simulink model "DEF_IEEE14_case2"  (R2022b)
settings: Solver=FixedStepAuto  StartTime=0  StopTime=60  FixedStep=Ts  RelTol=1e-3
StopFcn:
  | data_idq_all_case2 = out.data_idq_all_case2;
  | save('Oscillation_July\data\data_idq_all_case2.mat','data_idq_all_case2');
  | data_vdq_all_case2 = out.data_vdq_all_case2;
  | save('Oscillation_July\data\data_vdq_all_case2.mat','data_vdq_all_case2');
undefined symbols (not defined in the file or in its folder): ApparatusDiscreDamping, ApparatusPara, ApparatusPowerFlow, ApparatusType, Fbase, OtherInputs, Sbase, Ts, Vbase, Wbase, x_e, Ybase, Zbase
libraries: spsGroundLib x22, SimplusGT x22, spsThreePhaseSeriesRLCBranchLib x20, spsThreePhaseParallelRLCBranchLib x14, spsabctoAlphaBetaZeroLib x8, spsThreePhaseTransformerTwoWindingsLib x3, spspowerguiLib x1
(part 1 of 2)
settings Model: LastModifiedBy=y_zhu

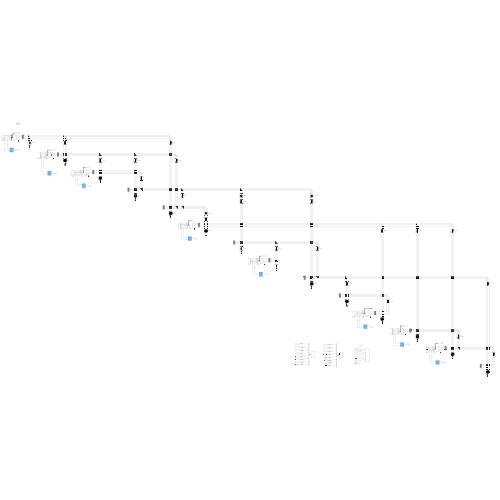
[thumbnail: Simulink's stored preview of the top-level diagram]
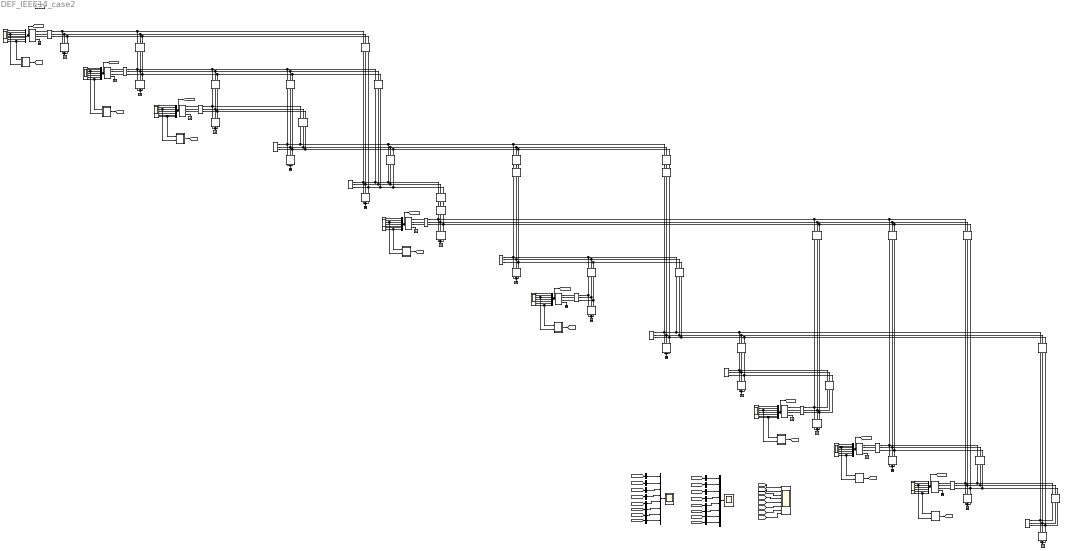
== system DEF_IEEE14_case2 ==
  note: DEF METHOD
  B-GND{1,4,8,10,14,16,20,23..24,27,29..30,32,34} (14 alike) : spsGroundLib/Ground  LConnTagsString=a
  Branch1-1 : spsThreePhaseParallelRLCBranchLib/Three-Phase Parallel RLC Branch  LConnTagsString=A|B|C  RConnTagsString=A|B|C  BranchType=C  Resistance=(Inf)*Zbase  Inductance=(Inf)*Zbase/Wbase  Capacitance=(0.051)*Ybase/Wbase  Measurements=None
  Branch1-2 : spsThreePhaseSeriesRLCBranchLib/Three-Phase Series RLC Branch  LConnTagsString=A|B|C  RConnTagsString=A|B|C  BranchType=RL  Resistance=(0.01938)*Zbase  Inductance=(0.05917)*Zbase/Wbase  Capacitance=1e-6  Measurements=None
  Branch1-5 : spsThreePhaseSeriesRLCBranchLib/Three-Phase Series RLC Branch  LConnTagsString=A|B|C  RConnTagsString=A|B|C  BranchType=RL  Resistance=(0.05403)*Zbase  Inductance=(0.22304)*Zbase/Wbase  Capacitance=1e-6  Measurements=None
  Branch10-10 : spsThreePhaseParallelRLCBranchLib/Three-Phase Parallel RLC Branch  LConnTagsString=A|B|C  RConnTagsString=A|B|C  BranchType=RLC  Resistance=(11.6045)*Zbase  Inductance=(18.007)*Zbase/Wbase  Capacitance=(1e-07)*Ybase/Wbase  Measurements=None
  Branch10-11 : spsThreePhaseSeriesRLCBranchLib/Three-Phase Series RLC Branch  LConnTagsString=A|B|C  RConnTagsString=A|B|C  BranchType=RL  Resistance=(0.08205)*Zbase  Inductance=(0.19207)*Zbase/Wbase  Capacitance=1e-6  Measurements=None
  Branch11-11 : spsThreePhaseParallelRLCBranchLib/Three-Phase Parallel RLC Branch  LConnTagsString=A|B|C  RConnTagsString=A|B|C  BranchType=RLC  Resistance=(11.2405)*Zbase  Inductance=(65.5695)*Zbase/Wbase  Capacitance=(1e-07)*Ybase/Wbase  Measurements=None
  Branch12-12 : spsThreePhaseParallelRLCBranchLib/Three-Phase Parallel RLC Branch  LConnTagsString=A|B|C  RConnTagsString=A|B|C  BranchType=RLC  Resistance=(7.226)*Zbase  Inductance=(82.6479)*Zbase/Wbase  Capacitance=(1e-07)*Ybase/Wbase  Measurements=None
  Branch12-13 : spsThreePhaseSeriesRLCBranchLib/Three-Phase Series RLC Branch  LConnTagsString=A|B|C  RConnTagsString=A|B|C  BranchType=RL  Resistance=(0.22092)*Zbase  Inductance=(0.19988)*Zbase/Wbase  Capacitance=1e-6  Measurements=None
  Branch13-13 : spsThreePhaseParallelRLCBranchLib/Three-Phase Parallel RLC Branch  LConnTagsString=A|B|C  RConnTagsString=A|B|C  BranchType=RLC  Resistance=(2.9586)*Zbase  Inductance=(20.6593)*Zbase/Wbase  Capacitance=(1.5e-07)*Ybase/Wbase  Measurements=None
  Branch13-14 : spsThreePhaseSeriesRLCBranchLib/Three-Phase Series RLC Branch  LConnTagsString=A|B|C  RConnTagsString=A|B|C  BranchType=RL  Resistance=(0.17093)*Zbase  Inductance=(0.34802)*Zbase/Wbase  Capacitance=1e-6  Measurements=None
  Branch14-14 : spsThreePhaseParallelRLCBranchLib/Three-Phase Parallel RLC Branch  LConnTagsString=A|B|C  RConnTagsString=A|B|C  BranchType=RLC  Resistance=(6.9827)*Zbase  Inductance=(20.8085)*Zbase/Wbase  Capacitance=(1e-07)*Ybase/Wbase  Measurements=None
  Branch2-2 : spsThreePhaseParallelRLCBranchLib/Three-Phase Parallel RLC Branch  LConnTagsString=A|B|C  RConnTagsString=A|B|C  BranchType=RLC  Resistance=(5.0324)*Zbase  Inductance=(8.5986)*Zbase/Wbase  Capacitance=(0.0826)*Ybase/Wbase  Measurements=None
  Branch2-3 : spsThreePhaseSeriesRLCBranchLib/Three-Phase Series RLC Branch  LConnTagsString=A|B|C  RConnTagsString=A|B|C  BranchType=RL  Resistance=(0.04699)*Zbase  Inductance=(0.19797)*Zbase/Wbase  Capacitance=1e-6  Measurements=None
  Branch2-4 : spsThreePhaseSeriesRLCBranchLib/Three-Phase Series RLC Branch  LConnTagsString=A|B|C  RConnTagsString=A|B|C  BranchType=RL  Resistance=(0.05811)*Zbase  Inductance=(0.17632)*Zbase/Wbase  Capacitance=1e-6  Measurements=None
  Branch2-5 : spsThreePhaseSeriesRLCBranchLib/Three-Phase Series RLC Branch  LConnTagsString=A|B|C  RConnTagsString=A|B|C  BranchType=RL  Resistance=(0.05695)*Zbase  Inductance=(0.17388)*Zbase/Wbase  Capacitance=1e-6  Measurements=None
  Branch3-3 : spsThreePhaseParallelRLCBranchLib/Three-Phase Parallel RLC Branch  LConnTagsString=A|B|C  RConnTagsString=A|B|C  BranchType=RLC  Resistance=(1.0792)*Zbase  Inductance=(5.3506)*Zbase/Wbase  Capacitance=(0.0283)*Ybase/Wbase  Measurements=None
  Branch3-4 : spsThreePhaseSeriesRLCBranchLib/Three-Phase Series RLC Branch  LConnTagsString=A|B|C  RConnTagsString=A|B|C  BranchType=RL  Resistance=(0.06701)*Zbase  Inductance=(0.17103)*Zbase/Wbase  Capacitance=1e-6  Measurements=None
  Branch4-4 : spsThreePhaseParallelRLCBranchLib/Three-Phase Parallel RLC Branch  LConnTagsString=A|B|C  RConnTagsString=A|B|C  BranchType=RC  Resistance=(2.232)*Zbase  Inductance=(Inf)*Zbase/Wbase  Capacitance=(0.059954)*Ybase/Wbase  Measurements=None
  Branch4-5 : spsThreePhaseSeriesRLCBranchLib/Three-Phase Series RLC Branch  LConnTagsString=A|B|C  RConnTagsString=A|B|C  BranchType=RL  Resistance=(0.01335)*Zbase  Inductance=(0.04211)*Zbase/Wbase  Capacitance=1e-6  Measurements=None
  Branch4-7 : spsThreePhaseSeriesRLCBranchLib/Three-Phase Series RLC Branch  LConnTagsString=A|B|C  RConnTagsString=A|B|C  BranchType=RL  Resistance=(1e-07)*Zbase  Inductance=(0.20912)*Zbase/Wbase  Capacitance=1e-6  Measurements=None
  Branch4-9 : spsThreePhaseSeriesRLCBranchLib/Three-Phase Series RLC Branch  LConnTagsString=A|B|C  RConnTagsString=A|B|C  BranchType=RL  Resistance=(1e-07)*Zbase  Inductance=(0.55618)*Zbase/Wbase  Capacitance=1e-6  Measurements=None
  Branch5-5 : spsThreePhaseParallelRLCBranchLib/Three-Phase Parallel RLC Branch  LConnTagsString=A|B|C  RConnTagsString=A|B|C  BranchType=RLC  Resistance=(14.1668)*Zbase  Inductance=(67.2925)*Zbase/Wbase  Capacitance=(0.0419)*Ybase/Wbase  Measurements=None
  Branch5-6 : spsThreePhaseSeriesRLCBranchLib/Three-Phase Series RLC Branch  LConnTagsString=A|B|C  RConnTagsString=A|B|C  BranchType=RL  Resistance=(1e-07)*Zbase  Inductance=(0.25202)*Zbase/Wbase  Capacitance=1e-6  Measurements=None
  Branch6-11 : spsThreePhaseSeriesRLCBranchLib/Three-Phase Series RLC Branch  LConnTagsString=A|B|C  RConnTagsString=A|B|C  BranchType=RL  Resistance=(0.09498)*Zbase  Inductance=(0.1989)*Zbase/Wbase  Capacitance=1e-6  Measurements=None
  Branch6-12 : spsThreePhaseSeriesRLCBranchLib/Three-Phase Series RLC Branch  LConnTagsString=A|B|C  RConnTagsString=A|B|C  BranchType=RL  Resistance=(0.12291)*Zbase  Inductance=(0.25581)*Zbase/Wbase  Capacitance=1e-6  Measurements=None
  Branch6-13 : spsThreePhaseSeriesRLCBranchLib/Three-Phase Series RLC Branch  LConnTagsString=A|B|C  RConnTagsString=A|B|C  BranchType=RL  Resistance=(0.06615)*Zbase  Inductance=(0.13027)*Zbase/Wbase  Capacitance=1e-6  Measurements=None
  Branch6-6 : spsThreePhaseParallelRLCBranchLib/Three-Phase Parallel RLC Branch  LConnTagsString=A|B|C  RConnTagsString=A|B|C  BranchType=RLC  Resistance=(10.2223)*Zbase  Inductance=(15.2653)*Zbase/Wbase  Capacitance=(2e-07)*Ybase/Wbase  Measurements=None
  Branch7-7 : spsThreePhaseParallelRLCBranchLib/Three-Phase Parallel RLC Branch  LConnTagsString=A|B|C  RConnTagsString=A|B|C  BranchType=C  Resistance=(Inf)*Zbase  Inductance=(Inf)*Zbase/Wbase  Capacitance=(1.5e-07)*Ybase/Wbase  Measurements=None
  Branch7-8 : spsThreePhaseSeriesRLCBranchLib/Three-Phase Series RLC Branch  LConnTagsString=A|B|C  RConnTagsString=A|B|C  BranchType=RL  Resistance=(1e-07)*Zbase  Inductance=(0.17615)*Zbase/Wbase  Capacitance=1e-6  Measurements=None
  Branch7-9 : spsThreePhaseSeriesRLCBranchLib/Three-Phase Series RLC Branch  LConnTagsString=A|B|C  RConnTagsString=A|B|C  BranchType=RL  Resistance=(1e-07)*Zbase  Inductance=(0.11001)*Zbase/Wbase  Capacitance=1e-6  Measurements=None
  Branch8-8 : spsThreePhaseParallelRLCBranchLib/Three-Phase Parallel RLC Branch  LConnTagsString=A|B|C  RConnTagsString=A|B|C  BranchType=C  Resistance=(Inf)*Zbase  Inductance=(Inf)*Zbase/Wbase  Capacitance=(5e-08)*Ybase/Wbase  Measurements=None
  Branch9-10 : spsThreePhaseSeriesRLCBranchLib/Three-Phase Series RLC Branch  LConnTagsString=A|B|C  RConnTagsString=A|B|C  BranchType=RL  Resistance=(0.03181)*Zbase  Inductance=(0.0845)*Zbase/Wbase  Capacitance=1e-6  Measurements=None
  Branch9-14 : spsThreePhaseSeriesRLCBranchLib/Three-Phase Series RLC Branch  LConnTagsString=A|B|C  RConnTagsString=A|B|C  BranchType=RL  Resistance=(0.12711)*Zbase  Inductance=(0.27038)*Zbase/Wbase  Capacitance=1e-6  Measurements=None
  Branch9-9 : spsThreePhaseParallelRLCBranchLib/Three-Phase Parallel RLC Branch  LConnTagsString=A|B|C  RConnTagsString=A|B|C  BranchType=RLC  Resistance=(3.4827)*Zbase  Inductance=(6.1892)*Zbase/Wbase  Capacitance=(0.19)*Ybase/Wbase  Measurements=None
  Bus Creator1 : BusCreator  Inputs=8
  Bus Creator2 : BusCreator  Inputs=8
  Bus Selector{,1..7} (8 alike) : BusSelector  OutputSignals=v_dq
  Bus Selector{8..15} (8 alike) : BusSelector  OutputSignals=i_dq
  Bus{1..14} (14 alike) : SimplusGT/Three-Phase Bus  Vbase=1  Sbase=1
      settings: SourceProductName=Simplus Grid Tool
  D-GND{1..3,6,8,11..13} (8 alike) : spsGroundLib/Ground  LConnTagsString=a
  D-Scope{1..3,6,8,11..13} (8 alike) : Scope  NumInputPorts=7
  DEF_Friction1 : Subsystem  mask{PowerFlow_App=ApparatusPowerFlow{2}, Tinit=10}
      mask prompts: PowerFlow_App "Power Flow"; Tinit "Initial Filter Time"
  DEF_Friction2 : Subsystem  mask{PowerFlow_App=ApparatusPowerFlow{3}, Tinit=10}
      mask prompts: PowerFlow_App "Power Flow"; Tinit "Initial Filter Time"
  DEF_Friction3 : Subsystem  mask{PowerFlow_App=ApparatusPowerFlow{1}, Tinit=10}
      mask prompts: PowerFlow_App "Power Flow"; Tinit "Initial Filter Time"
  DEF_Friction4 : Subsystem  mask{PowerFlow_App=ApparatusPowerFlow{6}, Tinit=10}
      mask prompts: PowerFlow_App "Power Flow"; Tinit "Initial Filter Time"
  DEF_Friction5 : Subsystem  mask{PowerFlow_App=ApparatusPowerFlow{8}, Tinit=10}
      mask prompts: PowerFlow_App "Power Flow"; Tinit "Initial Filter Time"
  DEF_Friction6 : Subsystem  mask{PowerFlow_App=ApparatusPowerFlow{11}, Tinit=10}
      mask prompts: PowerFlow_App "Power Flow"; Tinit "Initial Filter Time"
  DEF_Friction7 : Subsystem  mask{PowerFlow_App=ApparatusPowerFlow{12}, Tinit=10}
      mask prompts: PowerFlow_App "Power Flow"; Tinit "Initial Filter Time"
  DEF_Friction8 : Subsystem  mask{PowerFlow_App=ApparatusPowerFlow{13}, Tinit=10}
      mask prompts: PowerFlow_App "Power Flow"; Tinit "Initial Filter Time"
  DS-Bus{1..3,6,8,11..13} (8 alike) : BusSelector  OutputSignals=v_dq,i_dq,v_abc,i_abc,w,theta,pq
  SM1 : SimplusGT/SynchronousMachineFull_Cyp_SMAVRPSSGOV (dq-Frame System Object)  Ts=Ts  Sbase=Sbase  Vbase=Vbase  Wbase=Wbase  ApparatusType=ApparatusType{1}  ApparatusPara=ApparatusPara{1}  PowerFlow=ApparatusPowerFlow{1}  x0=x_e{1}  OtherInputs=OtherInputs{1}  DiscreMethod=Hybrid Trapezoidal  EnableInsideModification=off  DiscreDampingFlag=on  DiscreDampingValue=ApparatusDiscreDamping{1}  LinearizationTimes=1  DirectFeedthrough=off
      settings: SourceProductName=Simplus Grid Tool
  SM2 : SimplusGT/SynchronousMachineFull_Cyp_SMAVRPSSGOV (dq-Frame System Object)  Ts=Ts  Sbase=Sbase  Vbase=Vbase  Wbase=Wbase  ApparatusType=ApparatusType{2}  ApparatusPara=ApparatusPara{2}  PowerFlow=ApparatusPowerFlow{2}  x0=x_e{2}  OtherInputs=OtherInputs{2}  DiscreMethod=Hybrid Trapezoidal  EnableInsideModification=off  DiscreDampingFlag=on  DiscreDampingValue=ApparatusDiscreDamping{2}  LinearizationTimes=1  DirectFeedthrough=off
      settings: SourceProductName=Simplus Grid Tool
  SM3 : SimplusGT/SynchronousMachineFull_Cyp_SMAVR (dq-Frame System Object)  Ts=Ts  Sbase=Sbase  Vbase=Vbase  Wbase=Wbase  ApparatusType=ApparatusType{3}  ApparatusPara=ApparatusPara{3}  PowerFlow=ApparatusPowerFlow{3}  x0=x_e{3}  OtherInputs=OtherInputs{3}  DiscreMethod=Hybrid Trapezoidal  EnableInsideModification=off  DiscreDampingFlag=on  DiscreDampingValue=ApparatusDiscreDamping{3}  LinearizationTimes=1  DirectFeedthrough=off
      settings: SourceProductName=Simplus Grid Tool
  SM6 : SimplusGT/SynchronousMachineFull_Cyp_SMAVR (dq-Frame System Object)  Ts=Ts  Sbase=Sbase  Vbase=Vbase  Wbase=Wbase  ApparatusType=ApparatusType{6}  ApparatusPara=ApparatusPara{6}  PowerFlow=ApparatusPowerFlow{6}  x0=x_e{6}  OtherInputs=OtherInputs{6}  DiscreMethod=Hybrid Trapezoidal  EnableInsideModification=off  DiscreDampingFlag=on  DiscreDampingValue=ApparatusDiscreDamping{6}  LinearizationTimes=1  DirectFeedthrough=off
      settings: SourceProductName=Simplus Grid Tool
  SM8 : SimplusGT/SynchronousMachineFull_Cyp_SMAVR (dq-Frame System Object)  Ts=Ts  Sbase=Sbase  Vbase=Vbase  Wbase=Wbase  ApparatusType=ApparatusType{8}  ApparatusPara=ApparatusPara{8}  PowerFlow=ApparatusPowerFlow{8}  x0=x_e{8}  OtherInputs=OtherInputs{8}  DiscreMethod=Hybrid Trapezoidal  EnableInsideModification=off  DiscreDampingFlag=on  DiscreDampingValue=ApparatusDiscreDamping{8}  LinearizationTimes=1  DirectFeedthrough=off
      settings: SourceProductName=Simplus Grid Tool
  Scope : Scope  NumInputPorts=8
  Scope1 : Scope
  Scope7 : Scope
  Transformer4-7 : spsThreePhaseTransformerTwoWindingsLib/Three-Phase Transformer (Two Windings)  Winding1Connection=Yg  Winding2Connection=Yg  CoreType=Three single-phase transformers  SetSaturation=off  Hysteresis=off  DataFile='hysteresis'  SetInitialFlux=off  Measurements=None  UNITS=pu  NominalPower=[Sbase, Fbase]  Winding1=[0.978*Vbase, 0, 0]  Winding2=[Vbase, 0, 0]  Rm=1e4  Lm=1e4  L0=0.5  Saturation=[ 0,0 ; 0.0024,1.2 ; 1.0,1.52 ]  InitialFluxes=[ 0.8 , -0.8 , 0.7 ]  BreakLoop=off  DiscreteSolver=Trapezoidal iterative  DataType=off  TransfoNumber=1
  Transformer4-9 : spsThreePhaseTransformerTwoWindingsLib/Three-Phase Transformer (Two Windings)  Winding1Connection=Yg  Winding2Connection=Yg  CoreType=Three single-phase transformers  SetSaturation=off  Hysteresis=off  DataFile='hysteresis'  SetInitialFlux=off  Measurements=None  UNITS=pu  NominalPower=[Sbase, Fbase]  Winding1=[0.969*Vbase, 0, 0]  Winding2=[Vbase, 0, 0]  Rm=1e4  Lm=1e4  L0=0.5  Saturation=[ 0,0 ; 0.0024,1.2 ; 1.0,1.52 ]  InitialFluxes=[ 0.8 , -0.8 , 0.7 ]  BreakLoop=off  DiscreteSolver=Trapezoidal iterative  DataType=off  TransfoNumber=1
  Transformer5-6 : spsThreePhaseTransformerTwoWindingsLib/Three-Phase Transformer (Two Windings)  Winding1Connection=Yg  Winding2Connection=Yg  CoreType=Three single-phase transformers  SetSaturation=off  Hysteresis=off  DataFile='hysteresis'  SetInitialFlux=off  Measurements=None  UNITS=pu  NominalPower=[Sbase, Fbase]  Winding1=[0.932*Vbase, 0, 0]  Winding2=[Vbase, 0, 0]  Rm=1e4  Lm=1e4  L0=0.5  Saturation=[ 0,0 ; 0.0024,1.2 ; 1.0,1.52 ]  InitialFluxes=[ 0.8 , -0.8 , 0.7 ]  BreakLoop=off  DiscreteSolver=Trapezoidal iterative  DataType=off  TransfoNumber=1
  VSI-PLL11 : SimplusGT/Grid-Following Voltage-Source Inverter (dq-Frame System Object)  Ts=Ts  Sbase=Sbase  Vbase=Vbase  Wbase=Wbase  ApparatusType=ApparatusType{11}  ApparatusPara=ApparatusPara{11}  PowerFlow=ApparatusPowerFlow{11}  x0=x_e{11}  OtherInputs=OtherInputs{11}  DiscreMethod=Hybrid Trapezoidal  EnableInsideModification=off  DiscreDampingFlag=on  DiscreDampingValue=ApparatusDiscreDamping{11}  LinearizationTimes=1  DirectFeedthrough=off
      settings: SourceProductName=Simplus Grid Tool
  VSI-PLL12 : SimplusGT/Grid-Following Voltage-Source Inverter (dq-Frame System Object)  Ts=Ts  Sbase=Sbase  Vbase=Vbase  Wbase=Wbase  ApparatusType=ApparatusType{12}  ApparatusPara=ApparatusPara{12}  PowerFlow=ApparatusPowerFlow{12}  x0=x_e{12}  OtherInputs=OtherInputs{12}  DiscreMethod=Hybrid Trapezoidal  EnableInsideModification=off  DiscreDampingFlag=on  DiscreDampingValue=ApparatusDiscreDamping{12}  LinearizationTimes=1  DirectFeedthrough=off
      settings: SourceProductName=Simplus Grid Tool
  VSI-PLL13 : SimplusGT/Grid-Following Voltage-Source Inverter (dq-Frame System Object)  Ts=Ts  Sbase=Sbase  Vbase=Vbase  Wbase=Wbase  ApparatusType=ApparatusType{13}  ApparatusPara=ApparatusPara{13}  PowerFlow=ApparatusPowerFlow{13}  x0=x_e{13}  OtherInputs=OtherInputs{13}  DiscreMethod=Hybrid Trapezoidal  EnableInsideModification=off  DiscreDampingFlag=on  DiscreDampingValue=ApparatusDiscreDamping{13}  LinearizationTimes=1  DirectFeedthrough=off
      settings: SourceProductName=Simplus Grid Tool
  powergui : spspowerguiLib/powergui  Priority=1  SimulationMode=Discrete  SampleTime=Ts  frequency=60  Iterations=50  frequencyindice=0  Pbase=100e6  ErrMax=1e-4  UnitsV=kV  UnitsW=MW  buscounter=0  FunctionMessages=off  echomessages=off  EnableUseOfTLC=off  CurrentSourceSwitches=off  DisableSnubberDevices=off  DisableRonSwitches=off  DisableVfSwitches=off  DisplayEquations=off  AutomaticDiscreteSolvers=off  SolverType=Tustin/Backward Euler (TBE)  Interpol=off  ExternalGateDelay=off  methode=off  Ts=100  x0status=blocks  SPID=on  SwTol=0  HookPort=off  NonlinearTolerance=1e-4  nMaxIteration=100  ContinueOnMaxIteration=off  RestoreLinks=warning  ResistiveCurrentMeasurement=off  Frange=[0:2:500]  Ylog=off  Xlog=on  ShowGrid=off  save=off  variable=ZData  structure=0  ZoomFFT=off  StartTime=0.0  cycles=1  DisplayStyle=1  fundamental=60  FreqAxis=off  MaxFrequency=1000  frequencyindicesteady=1  RmsSteady=1  display=off
  wires:
  DS-Bus1/1 -> D-Scope1/1  "<v_dq>"
  DS-Bus1/2 -> D-Scope1/2  "<i_dq>"
  DS-Bus1/4 -> D-Scope1/4  "<i_abc>"
  DS-Bus1/5 -> D-Scope1/5  "<w>"
  DS-Bus1/6 -> D-Scope1/6  "<theta>"
  DS-Bus2/1 -> D-Scope2/1  "<v_dq>"
  DS-Bus2/2 -> D-Scope2/2  "<i_dq>"
  DS-Bus2/4 -> D-Scope2/4  "<i_abc>"
  DS-Bus2/5 -> D-Scope2/5  "<w>"
  DS-Bus2/6 -> D-Scope2/6  "<theta>"
  DS-Bus3/1 -> D-Scope3/1  "<v_dq>"
  DS-Bus3/2 -> D-Scope3/2  "<i_dq>"
  DS-Bus3/4 -> D-Scope3/4  "<i_abc>"
  DS-Bus3/5 -> D-Scope3/5  "<w>"
  DS-Bus3/6 -> D-Scope3/6  "<theta>"
  DS-Bus6/1 -> D-Scope6/1  "<v_dq>"
  DS-Bus6/2 -> D-Scope6/2  "<i_dq>"
  DS-Bus6/4 -> D-Scope6/4  "<i_abc>"
  DS-Bus6/5 -> D-Scope6/5  "<w>"
  DS-Bus6/6 -> D-Scope6/6  "<theta>"
  DS-Bus8/1 -> D-Scope8/1  "<v_dq>"
  DS-Bus8/2 -> D-Scope8/2  "<i_dq>"
  DS-Bus8/4 -> D-Scope8/4  "<i_abc>"
  DS-Bus8/5 -> D-Scope8/5  "<w>"
  DS-Bus8/6 -> D-Scope8/6  "<theta>"
  DS-Bus11/1 -> D-Scope11/1  "<v_dq>"
  DS-Bus11/2 -> D-Scope11/2  "<i_dq>"
  DS-Bus11/4 -> D-Scope11/4  "<i_abc>"
  DS-Bus11/5 -> D-Scope11/5  "<w>"
  DS-Bus11/6 -> D-Scope11/6  "<theta>"
  DS-Bus12/1 -> D-Scope12/1  "<v_dq>"
  DS-Bus12/2 -> D-Scope12/2  "<i_dq>"
  DS-Bus12/4 -> D-Scope12/4  "<i_abc>"
  DS-Bus12/5 -> D-Scope12/5  "<w>"
  DS-Bus12/6 -> D-Scope12/6  "<theta>"
  DS-Bus13/1 -> D-Scope13/1  "<v_dq>"
  DS-Bus13/2 -> D-Scope13/2  "<i_dq>"
  DS-Bus13/4 -> D-Scope13/4  "<i_abc>"
  DS-Bus13/5 -> D-Scope13/5  "<w>"
  DS-Bus13/6 -> D-Scope13/6  "<theta>"
  DS-Bus1/7 -> DEF_Friction3/1(PQ), D-Scope1/7  "<pq>"
  DEF_Friction3/1(DEF) -> [A1]
  DS-Bus1/3 -> DEF_Friction3/2(Vabc), D-Scope1/3  "<v_abc>"
  DS-Bus2/7 -> DEF_Friction1/1(PQ), D-Scope2/7  "<pq>"
  DS-Bus2/3 -> DEF_Friction1/2(Vabc), D-Scope2/3  "<v_abc>"
  DEF_Friction1/1(DEF) -> [A2]
  DS-Bus3/7 -> DEF_Friction2/1(PQ), D-Scope3/7  "<pq>"
  DEF_Friction2/1(DEF) -> [A3]
  DS-Bus3/3 -> DEF_Friction2/2(Vabc), D-Scope3/3  "<v_abc>"
  DEF_Friction4/1(DEF) -> [A6]
  DS-Bus6/3 -> DEF_Friction4/2(Vabc), D-Scope6/3  "<v_abc>"
  DS-Bus6/7 -> DEF_Friction4/1(PQ), D-Scope6/7  "<pq>"
  DEF_Friction5/1(DEF) -> [A8]
  DS-Bus8/3 -> DEF_Friction5/2(Vabc), D-Scope8/3  "<v_abc>"
  DS-Bus8/7 -> DEF_Friction5/1(PQ), D-Scope8/7  "<pq>"
  DEF_Friction6/1(DEF) -> [A11]
  DS-Bus11/3 -> DEF_Friction6/2(Vabc), D-Scope11/3  "<v_abc>"
  DS-Bus11/7 -> DEF_Friction6/1(PQ), D-Scope11/7  "<pq>"
  DEF_Friction7/1(DEF) -> [A12]
  DS-Bus12/3 -> DEF_Friction7/2(Vabc), D-Scope12/3  "<v_abc>"
  DS-Bus12/7 -> DEF_Friction7/1(PQ), D-Scope12/7  "<pq>"
  DS-Bus13/7 -> DEF_Friction8/1(PQ), D-Scope13/7  "<pq>"
  DEF_Friction8/1(DEF) -> [A13]
  DS-Bus13/3 -> DEF_Friction8/2(Vabc), D-Scope13/3  "<v_abc>"
  [A1] -> Scope/1  "A1"
  [A2] -> Scope/2  "A2"
  [A3] -> Scope/3  "A3"
  [A6] -> Scope/4  "A6"
  [A8] -> Scope/5  "A8"
  [A11] -> Scope/6  "A11"
  [A12] -> Scope/7  "A12"
  [A13] -> Scope/8  "A13"
  [A6_measure] -> Bus Selector3/1
  [A8_measure] -> Bus Selector4/1
  Bus Selector7/1 -> Bus Creator2/8  "<v_dq>"
  Bus Selector6/1 -> Bus Creator2/7  "<v_dq>"
  Bus Selector5/1 -> Bus Creator2/6  "<v_dq>"
  [A11_measure] -> Bus Selector5/1
  Bus Selector2/1 -> Bus Creator2/3  "<v_dq>"
  [A2_measure] -> Bus Selector1/1
  Bus Creator2/1 -> Scope7/1
  Bus Selector/1 -> Bus Creator2/1  "<v_dq>"
  Bus Selector3/1 -> Bus Creator2/4  "<v_dq>"
  [A12_measure] -> Bus Selector6/1
  Bus Selector1/1 -> Bus Creator2/2  "<v_dq>"
  [A3_measure] -> Bus Selector2/1
  [A1_measure] -> Bus Selector/1
  [A13_measure] -> Bus Selector7/1
  Bus Selector4/1 -> Bus Creator2/5  "<v_dq>"
  VSI-PLL13/1 -> [A13_measure], DS-Bus13/1
  VSI-PLL12/1 -> [A12_measure], DS-Bus12/1
  VSI-PLL11/1 -> [A11_measure], DS-Bus11/1
  SM8/1 -> [A8_measure], DS-Bus8/1
  SM6/1 -> [A6_measure], DS-Bus6/1
  SM3/1 -> [A3_measure], DS-Bus3/1
  SM2/1 -> [A2_measure], DS-Bus2/1
  SM1/1 -> [A1_measure], DS-Bus1/1
  [A13_measure] -> Bus Selector15/1
  [A1_measure] -> Bus Selector8/1
  [A3_measure] -> Bus Selector10/1
  Bus Selector12/1 -> Bus Creator1/5  "<i_dq>"
  Bus Selector13/1 -> Bus Creator1/6  "<i_dq>"
  Bus Selector10/1 -> Bus Creator1/3  "<i_dq>"
  [A12_measure] -> Bus Selector14/1
  Bus Selector14/1 -> Bus Creator1/7  "<i_dq>"
  [A2_measure] -> Bus Selector9/1
  [A11_measure] -> Bus Selector13/1
  Bus Selector11/1 -> Bus Creator1/4  "<i_dq>"
  Bus Selector15/1 -> Bus Creator1/8  "<i_dq>"
  Bus Selector8/1 -> Bus Creator1/1  "<i_dq>"
  Bus Selector9/1 -> Bus Creator1/2  "<i_dq>"
  [A8_measure] -> Bus Selector12/1
  [A6_measure] -> Bus Selector11/1
  Bus Creator1/1 -> Scope1/1
  connections:
  SM1/LConn4 -- D-GND1/LConn1
  SM2/LConn4 -- D-GND2/LConn1
  SM3/LConn4 -- D-GND3/LConn1
  SM6/LConn4 -- D-GND6/LConn1
  SM8/LConn4 -- D-GND8/LConn1
  VSI-PLL11/LConn4 -- D-GND11/LConn1
  VSI-PLL12/LConn4 -- D-GND12/LConn1
  VSI-PLL13/LConn4 -- D-GND13/LConn1
  Branch1-1/RConn1 -- Branch1-1/RConn2 -- Branch1-1/RConn3 -- B-GND1/LConn1
  Branch2-2/RConn1 -- Branch2-2/RConn2 -- Branch2-2/RConn3 -- B-GND4/LConn1
  Branch3-3/RConn1 -- Branch3-3/RConn2 -- Branch3-3/RConn3 -- B-GND8/LConn1
  Branch4-4/RConn1 -- Branch4-4/RConn2 -- Branch4-4/RConn3 -- B-GND10/LConn1
  Branch5-5/RConn1 -- Branch5-5/RConn2 -- Branch5-5/RConn3 -- B-GND14/LConn1
  Branch6-6/RConn1 -- Branch6-6/RConn2 -- Branch6-6/RConn3 -- B-GND16/LConn1
  Branch7-7/RConn1 -- Branch7-7/RConn2 -- Branch7-7/RConn3 -- B-GND20/LConn1
  Branch8-8/RConn1 -- Branch8-8/RConn2 -- Branch8-8/RConn3 -- B-GND23/LConn1
  Branch9-9/RConn1 -- Branch9-9/RConn2 -- Branch9-9/RConn3 -- B-GND24/LConn1
  Branch10-10/RConn1 -- Branch10-10/RConn2 -- Branch10-10/RConn3 -- B-GND27/LConn1
  Branch11-11/RConn1 -- Branch11-11/RConn2 -- Branch11-11/RConn3 -- B-GND29/LConn1
  Branch12-12/RConn1 -- Branch12-12/RConn2 -- Branch12-12/RConn3 -- B-GND30/LConn1
  Branch13-13/RConn1 -- Branch13-13/RConn2 -- Branch13-13/RConn3 -- B-GND32/LConn1
  Branch14-14/RConn1 -- Branch14-14/RConn2 -- Branch14-14/RConn3 -- B-GND34/LConn1
  Branch1-2/RConn1 -- Bus2/RConn1 -- Branch2-2/LConn1 -- Branch2-5/LConn1 -- Branch2-4/LConn1 -- Branch2-3/LConn1
  Branch1-2/RConn2 -- Bus2/RConn2 -- Branch2-2/LConn2 -- Branch2-5/LConn2 -- Branch2-4/LConn2 -- Branch2-3/LConn2
  Branch1-2/RConn3 -- Bus2/RConn3 -- Branch2-2/LConn3 -- Branch2-5/LConn3 -- Branch2-4/LConn3 -- Branch2-3/LConn3
  Branch1-2/LConn1 -- Bus1/RConn1 -- Branch1-1/LConn1 -- Branch1-5/LConn1
  Branch1-2/LConn2 -- Bus1/RConn2 -- Branch1-1/LConn2 -- Branch1-5/LConn2
  Branch1-2/LConn3 -- Bus1/RConn3 -- Branch1-1/LConn3 -- Branch1-5/LConn3
  Branch1-5/RConn1 -- Bus5/RConn1 -- Branch5-5/LConn1 -- Transformer5-6/LConn1 -- Branch4-5/RConn1 -- Branch2-5/RConn1
  Branch1-5/RConn2 -- Bus5/RConn2 -- Branch5-5/LConn2 -- Transformer5-6/LConn2 -- Branch4-5/RConn2 -- Branch2-5/RConn2
  Branch1-5/RConn3 -- Bus5/RConn3 -- Branch5-5/LConn3 -- Transformer5-6/LConn3 -- Branch4-5/RConn3 -- Branch2-5/RConn3
  Branch2-3/RConn1 -- Bus3/RConn1 -- Branch3-3/LConn1 -- Branch3-4/LConn1
  Branch2-3/RConn2 -- Bus3/RConn2 -- Branch3-3/LConn2 -- Branch3-4/LConn2
  Branch2-3/RConn3 -- Bus3/RConn3 -- Branch3-3/LConn3 -- Branch3-4/LConn3
  Branch2-4/RConn1 -- Bus4/RConn1 -- Branch4-4/LConn1 -- Transformer4-9/LConn1 -- Transformer4-7/LConn1 -- Branch4-5/LConn1 -- Branch3-4/RConn1
  Branch2-4/RConn2 -- Bus4/RConn2 -- Branch4-4/LConn2 -- Transformer4-9/LConn2 -- Transformer4-7/LConn2 -- Branch4-5/LConn2 -- Branch3-4/RConn2
  Branch2-4/RConn3 -- Bus4/RConn3 -- Branch4-4/LConn3 -- Transformer4-9/LConn3 -- Transformer4-7/LConn3 -- Branch4-5/LConn3 -- Branch3-4/RConn3
  Branch4-7/RConn1 -- Bus7/RConn1 -- Branch7-7/LConn1 -- Branch7-9/LConn1 -- Branch7-8/LConn1
  Branch4-7/RConn2 -- Bus7/RConn2 -- Branch7-7/LConn2 -- Branch7-9/LConn2 -- Branch7-8/LConn2
  Branch4-7/RConn3 -- Bus7/RConn3 -- Branch7-7/LConn3 -- Branch7-9/LConn3 -- Branch7-8/LConn3
  Transformer4-7/RConn1 -- Branch4-7/LConn1
  Transformer4-7/RConn2 -- Branch4-7/LConn2
  Transformer4-7/RConn3 -- Branch4-7/LConn3
  Branch4-9/RConn1 -- Bus9/RConn1 -- Branch9-9/LConn1 -- Branch9-14/LConn1 -- Branch9-10/LConn1 -- Branch7-9/RConn1
  Branch4-9/RConn2 -- Bus9/RConn2 -- Branch9-9/LConn2 -- Branch9-14/LConn2 -- Branch9-10/LConn2 -- Branch7-9/RConn2
  Branch4-9/RConn3 -- Bus9/RConn3 -- Branch9-9/LConn3 -- Branch9-14/LConn3 -- Branch9-10/LConn3 -- Branch7-9/RConn3
  Transformer4-9/RConn1 -- Branch4-9/LConn1
  Transformer4-9/RConn2 -- Branch4-9/LConn2
  Transformer4-9/RConn3 -- Branch4-9/LConn3
  Branch5-6/RConn1 -- Bus6/RConn1 -- Branch6-6/LConn1 -- Branch6-13/LConn1 -- Branch6-12/LConn1 -- Branch6-11/LConn1
  Branch5-6/RConn2 -- Bus6/RConn2 -- Branch6-6/LConn2 -- Branch6-13/LConn2 -- Branch6-12/LConn2 -- Branch6-11/LConn2
  Branch5-6/RConn3 -- Bus6/RConn3 -- Branch6-6/LConn3 -- Branch6-13/LConn3 -- Branch6-12/LConn3 -- Branch6-11/LConn3
  Transformer5-6/RConn1 -- Branch5-6/LConn1
  Transformer5-6/RConn2 -- Branch5-6/LConn2
  Transformer5-6/RConn3 -- Branch5-6/LConn3
  Branch6-11/RConn1 -- Bus11/RConn1 -- Branch11-11/LConn1 -- Branch10-11/RConn1
  Branch6-11/RConn2 -- Bus11/RConn2 -- Branch11-11/LConn2 -- Branch10-11/RConn2
  Branch6-11/RConn3 -- Bus11/RConn3 -- Branch11-11/LConn3 -- Branch10-11/RConn3
  Branch6-12/RConn1 -- Bus12/RConn1 -- Branch12-12/LConn1 -- Branch12-13/LConn1
  Branch6-12/RConn2 -- Bus12/RConn2 -- Branch12-12/LConn2 -- Branch12-13/LConn2
  Branch6-12/RConn3 -- Bus12/RConn3 -- Branch12-12/LConn3 -- Branch12-13/LConn3
  Branch6-13/RConn1 -- Bus13/RConn1 -- Branch13-13/LConn1 -- Branch13-14/LConn1 -- Branch12-13/RConn1
  Branch6-13/RConn2 -- Bus13/RConn2 -- Branch13-13/LConn2 -- Branch13-14/LConn2 -- Branch12-13/RConn2
  Branch6-13/RConn3 -- Bus13/RConn3 -- Branch13-13/LConn3 -- Branch13-14/LConn3 -- Branch12-13/RConn3
  Branch7-8/RConn1 -- Bus8/RConn1 -- Branch8-8/LConn1
  Branch7-8/RConn2 -- Bus8/RConn2 -- Branch8-8/LConn2
  Branch7-8/RConn3 -- Bus8/RConn3 -- Branch8-8/LConn3
  Branch9-10/RConn1 -- Bus10/RConn1 -- Branch10-10/LConn1 -- Branch10-11/LConn1
  Branch9-10/RConn2 -- Bus10/RConn2 -- Branch10-10/LConn2 -- Branch10-11/LConn2
  Branch9-10/RConn3 -- Bus10/RConn3 -- Branch10-10/LConn3 -- Branch10-11/LConn3
  Branch9-14/RConn1 -- Bus14/RConn1 -- Branch14-14/LConn1 -- Branch13-14/RConn1
  Branch9-14/RConn2 -- Bus14/RConn2 -- Branch14-14/LConn2 -- Branch13-14/RConn2
  Branch9-14/RConn3 -- Bus14/RConn3 -- Branch14-14/LConn3 -- Branch13-14/RConn3
  SM1/LConn1 -- Bus1/LConn1
  SM1/LConn2 -- Bus1/LConn2
  SM1/LConn3 -- Bus1/LConn3
  SM2/LConn1 -- Bus2/LConn1
  SM2/LConn2 -- Bus2/LConn2
  SM2/LConn3 -- Bus2/LConn3
  SM3/LConn1 -- Bus3/LConn1
  SM3/LConn2 -- Bus3/LConn2
  SM3/LConn3 -- Bus3/LConn3
  SM6/LConn1 -- Bus6/LConn1
  SM6/LConn2 -- Bus6/LConn2
  SM6/LConn3 -- Bus6/LConn3
  SM8/LConn1 -- Bus8/LConn1
  SM8/LConn2 -- Bus8/LConn2
  SM8/LConn3 -- Bus8/LConn3
  VSI-PLL11/LConn1 -- Bus11/LConn1
  VSI-PLL11/LConn2 -- Bus11/LConn2
  VSI-PLL11/LConn3 -- Bus11/LConn3
  VSI-PLL12/LConn1 -- Bus12/LConn1
  VSI-PLL12/LConn2 -- Bus12/LConn2
  VSI-PLL12/LConn3 -- Bus12/LConn3
  VSI-PLL13/LConn1 -- Bus13/LConn1
  VSI-PLL13/LConn2 -- Bus13/LConn2
  VSI-PLL13/LConn3 -- Bus13/LConn3

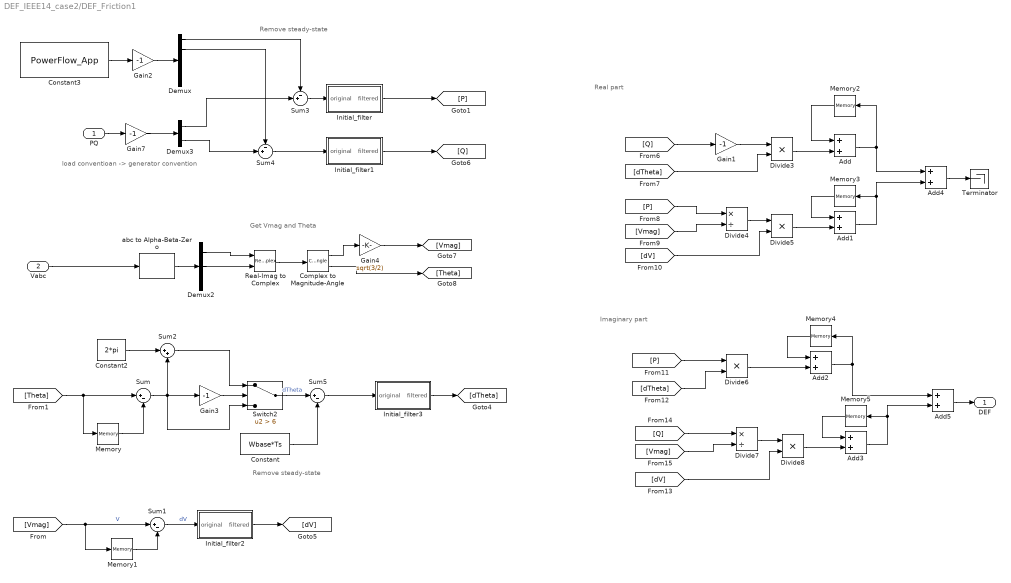
== system DEF_IEEE14_case2/DEF_Friction1 ==
  note: Real part
  note: Imaginary part
  note: load conventioan -> generator convention
  note: Remove steady-state
  note: Remove steady-state
  note: Get Vmag and Theta
  PQ : Inport
  Vabc : Inport  Port=2
  Add{,1..5} (6 alike) : Sum
  Complex to Magnitude-Angle : ComplexToMagnitudeAngle
  Constant : Constant  Value=Wbase*Ts
  Constant2 : Constant  Value=2*pi
  Constant3 : Constant  Value=PowerFlow_App
  Demux : Demux  Outputs=5
  Demux2 : Demux  Outputs=3
  Demux3 : Demux  Outputs=2
  Divide{3,5..6,8} (4 alike) : Product  Inputs=**
  Divide4 : Product  Inputs=*/
  Divide7 : Product  Inputs=*/
  Gain{1..3,7} (4 alike) : Gain  Gain=-1
  Gain4 : Gain  Gain=sqrt(3/2)
  Initial_filter : Subsystem
  Initial_filter1 : Subsystem
  Initial_filter2 : Subsystem
  Initial_filter3 : Subsystem
  Memory{,1..5} (6 alike) : Memory
  Real-Imag to Complex : RealImagToComplex
  Sum : Sum  Inputs=|+-
  Sum1 : Sum  Inputs=|+-
  Sum2 : Sum  Inputs=|++
  Sum3 : Sum  Inputs=-+|
  Sum4 : Sum  Inputs=-+|
  Sum5 : Sum  Inputs=|+-
  Switch2 : Switch  Criteria=u2 > Threshold  Threshold=6  SaturateOnIntegerOverflow=off  InputSameDT=off
  Terminator : Terminator
  abc to Alpha-Beta-Zero : spsabctoAlphaBetaZeroLib/abc to Alpha-Beta-Zero
  DEF : Outport
  wires:
  [Q] -> Divide7/1
  [Vmag] -> Divide4/2
  Divide3/1 -> Add/2
  [P] -> Divide4/1
  [Q] -> Gain1/1
  Gain1/1 -> Divide3/1
  [dTheta] -> Divide3/2
  [dV] -> Divide5/2
  [P] -> Divide6/1
  Divide4/1 -> Divide5/1
  [dTheta] -> Divide6/2
  [dV] -> Divide8/2
  Divide7/1 -> Divide8/1
  [Vmag] -> Divide7/2
  Memory1/1 -> Sum1/2
  [Vmag] -> Memory1/1, Sum1/1  "V"
  Sum1/1 -> Initial_filter2/1(original)  "dV"
  [Theta] -> Sum/1, Memory/1
  Add/1 -> Memory2/1, Add4/1
  Memory2/1 -> Add/1
  Divide5/1 -> Add1/2
  Add1/1 -> Add4/2, Memory3/1
  Memory3/1 -> Add1/1
  Memory4/1 -> Add2/1
  Add2/1 -> Add5/1, Memory4/1
  Divide6/1 -> Add2/2
  Memory5/1 -> Add3/1
  Add3/1 -> Add5/2, Memory5/1
  Divide8/1 -> Add3/2
  Vabc/1 -> abc to Alpha-Beta-Zero/1
  abc to Alpha-Beta-Zero/1 -> Demux2/1
  Memory/1 -> Sum/2
  Sum/1 -> Gain3/1, Switch2/3, Sum2/2
  Sum2/1 -> Switch2/1
  Constant2/1 -> Sum2/1
  Gain3/1 -> Switch2/2
  Constant3/1 -> Gain2/1
  Sum3/1 -> Initial_filter/1(original)
  Demux/1 -> Sum3/1
  Sum4/1 -> Initial_filter1/1(original)
  Demux/2 -> Sum4/1
  Demux3/1 -> Sum3/2
  Demux3/2 -> Sum4/2
  PQ/1 -> Gain7/1
  Initial_filter/1(filtered) -> [P]
  Initial_filter1/1(filtered) -> [Q]
  Initial_filter2/1(filtered) -> [dV]
  Initial_filter3/1(filtered) -> [dTheta]
  Complex to Magnitude-Angle/2 -> [Theta]
  Gain4/1 -> [Vmag]
  Complex to Magnitude-Angle/1 -> Gain4/1
  Real-Imag to Complex/1 -> Complex to Magnitude-Angle/1
  Demux2/1 -> Real-Imag to Complex/1
  Demux2/2 -> Real-Imag to Complex/2
  Gain2/1 -> Demux/1
  Gain7/1 -> Demux3/1
  Switch2/1 -> Sum5/1  "dTheta"
  Sum5/1 -> Initial_filter3/1(original)
  Constant/1 -> Sum5/2
  Add5/1 -> DEF/1
  Add4/1 -> Terminator/1

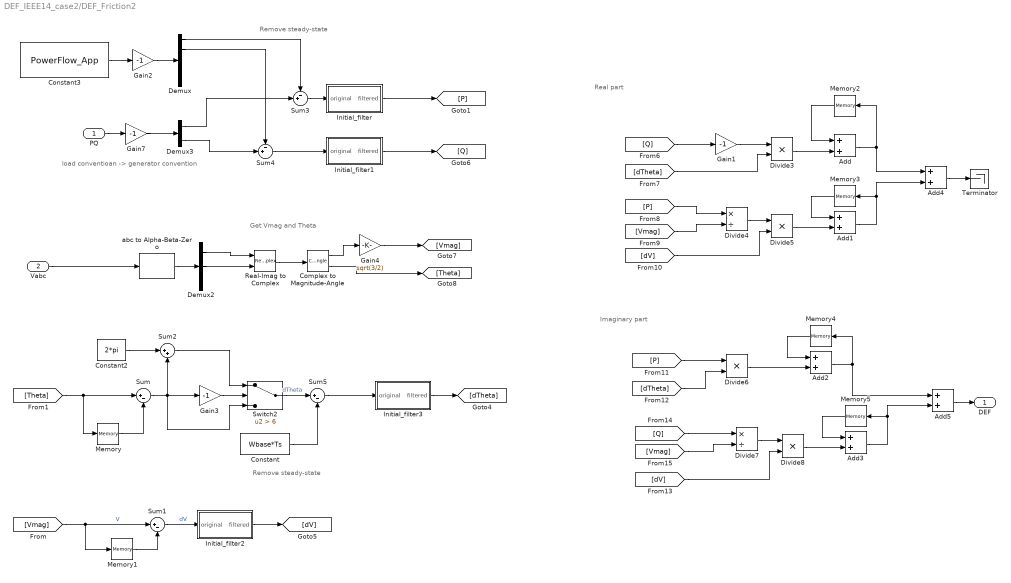
== system DEF_IEEE14_case2/DEF_Friction2 ==
  note: Real part
  note: Imaginary part
  note: load conventioan -> generator convention
  note: Remove steady-state
  note: Remove steady-state
  note: Get Vmag and Theta
  PQ : Inport
  Vabc : Inport  Port=2
  Add{,1..5} (6 alike) : Sum
  Complex to Magnitude-Angle : ComplexToMagnitudeAngle
  Constant : Constant  Value=Wbase*Ts
  Constant2 : Constant  Value=2*pi
  Constant3 : Constant  Value=PowerFlow_App
  Demux : Demux  Outputs=5
  Demux2 : Demux  Outputs=3
  Demux3 : Demux  Outputs=2
  Divide{3,5..6,8} (4 alike) : Product  Inputs=**
  Divide4 : Product  Inputs=*/
  Divide7 : Product  Inputs=*/
  Gain{1..3,7} (4 alike) : Gain  Gain=-1
  Gain4 : Gain  Gain=sqrt(3/2)
  Initial_filter : Subsystem
  Initial_filter1 : Subsystem
  Initial_filter2 : Subsystem
  Initial_filter3 : Subsystem
  Memory{,1..5} (6 alike) : Memory
  Real-Imag to Complex : RealImagToComplex
  Sum : Sum  Inputs=|+-
  Sum1 : Sum  Inputs=|+-
  Sum2 : Sum  Inputs=|++
  Sum3 : Sum  Inputs=-+|
  Sum4 : Sum  Inputs=-+|
  Sum5 : Sum  Inputs=|+-
  Switch2 : Switch  Criteria=u2 > Threshold  Threshold=6  SaturateOnIntegerOverflow=off  InputSameDT=off
  Terminator : Terminator
  abc to Alpha-Beta-Zero : spsabctoAlphaBetaZeroLib/abc to Alpha-Beta-Zero
  DEF : Outport
  wires:
  [Q] -> Divide7/1
  [Vmag] -> Divide4/2
  Divide3/1 -> Add/2
  [P] -> Divide4/1
  [Q] -> Gain1/1
  Gain1/1 -> Divide3/1
  [dTheta] -> Divide3/2
  [dV] -> Divide5/2
  [P] -> Divide6/1
  Divide4/1 -> Divide5/1
  [dTheta] -> Divide6/2
  [dV] -> Divide8/2
  Divide7/1 -> Divide8/1
  [Vmag] -> Divide7/2
  Memory1/1 -> Sum1/2
  [Vmag] -> Memory1/1, Sum1/1  "V"
  Sum1/1 -> Initial_filter2/1(original)  "dV"
  [Theta] -> Sum/1, Memory/1
  Add/1 -> Memory2/1, Add4/1
  Memory2/1 -> Add/1
  Divide5/1 -> Add1/2
  Add1/1 -> Add4/2, Memory3/1
  Memory3/1 -> Add1/1
  Memory4/1 -> Add2/1
  Add2/1 -> Add5/1, Memory4/1
  Divide6/1 -> Add2/2
  Memory5/1 -> Add3/1
  Add3/1 -> Add5/2, Memory5/1
  Divide8/1 -> Add3/2
  Vabc/1 -> abc to Alpha-Beta-Zero/1
  abc to Alpha-Beta-Zero/1 -> Demux2/1
  Memory/1 -> Sum/2
  Sum/1 -> Gain3/1, Switch2/3, Sum2/2
  Sum2/1 -> Switch2/1
  Constant2/1 -> Sum2/1
  Gain3/1 -> Switch2/2
  Constant3/1 -> Gain2/1
  Sum3/1 -> Initial_filter/1(original)
  Demux/1 -> Sum3/1
  Sum4/1 -> Initial_filter1/1(original)
  Demux/2 -> Sum4/1
  Demux3/1 -> Sum3/2
  Demux3/2 -> Sum4/2
  PQ/1 -> Gain7/1
  Initial_filter/1(filtered) -> [P]
  Initial_filter1/1(filtered) -> [Q]
  Initial_filter2/1(filtered) -> [dV]
  Initial_filter3/1(filtered) -> [dTheta]
  Complex to Magnitude-Angle/2 -> [Theta]
  Gain4/1 -> [Vmag]
  Complex to Magnitude-Angle/1 -> Gain4/1
  Real-Imag to Complex/1 -> Complex to Magnitude-Angle/1
  Demux2/1 -> Real-Imag to Complex/1
  Demux2/2 -> Real-Imag to Complex/2
  Gain2/1 -> Demux/1
  Gain7/1 -> Demux3/1
  Switch2/1 -> Sum5/1  "dTheta"
  Sum5/1 -> Initial_filter3/1(original)
  Constant/1 -> Sum5/2
  Add5/1 -> DEF/1
  Add4/1 -> Terminator/1

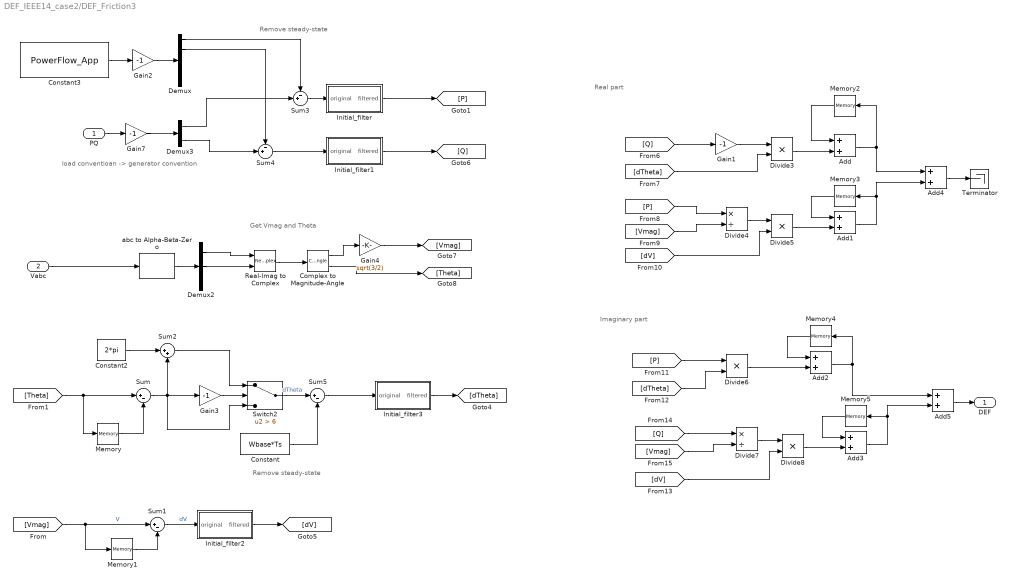
== system DEF_IEEE14_case2/DEF_Friction3 ==
  note: Real part
  note: Imaginary part
  note: load conventioan -> generator convention
  note: Remove steady-state
  note: Remove steady-state
  note: Get Vmag and Theta
  PQ : Inport
  Vabc : Inport  Port=2
  Add{,1..5} (6 alike) : Sum
  Complex to Magnitude-Angle : ComplexToMagnitudeAngle
  Constant : Constant  Value=Wbase*Ts
  Constant2 : Constant  Value=2*pi
  Constant3 : Constant  Value=PowerFlow_App
  Demux : Demux  Outputs=5
  Demux2 : Demux  Outputs=3
  Demux3 : Demux  Outputs=2
  Divide{3,5..6,8} (4 alike) : Product  Inputs=**
  Divide4 : Product  Inputs=*/
  Divide7 : Product  Inputs=*/
  Gain{1..3,7} (4 alike) : Gain  Gain=-1
  Gain4 : Gain  Gain=sqrt(3/2)
  Initial_filter : Subsystem
  Initial_filter1 : Subsystem
  Initial_filter2 : Subsystem
  Initial_filter3 : Subsystem
  Memory{,1..5} (6 alike) : Memory
  Real-Imag to Complex : RealImagToComplex
  Sum : Sum  Inputs=|+-
  Sum1 : Sum  Inputs=|+-
  Sum2 : Sum  Inputs=|++
  Sum3 : Sum  Inputs=-+|
  Sum4 : Sum  Inputs=-+|
  Sum5 : Sum  Inputs=|+-
  Switch2 : Switch  Criteria=u2 > Threshold  Threshold=6  SaturateOnIntegerOverflow=off  InputSameDT=off
  Terminator : Terminator
  abc to Alpha-Beta-Zero : spsabctoAlphaBetaZeroLib/abc to Alpha-Beta-Zero
  DEF : Outport
  wires:
  [Q] -> Divide7/1
  [Vmag] -> Divide4/2
  Divide3/1 -> Add/2
  [P] -> Divide4/1
  [Q] -> Gain1/1
  Gain1/1 -> Divide3/1
  [dTheta] -> Divide3/2
  [dV] -> Divide5/2
  [P] -> Divide6/1
  Divide4/1 -> Divide5/1
  [dTheta] -> Divide6/2
  [dV] -> Divide8/2
  Divide7/1 -> Divide8/1
  [Vmag] -> Divide7/2
  Memory1/1 -> Sum1/2
  [Vmag] -> Memory1/1, Sum1/1  "V"
  Sum1/1 -> Initial_filter2/1(original)  "dV"
  [Theta] -> Sum/1, Memory/1
  Add/1 -> Memory2/1, Add4/1
  Memory2/1 -> Add/1
  Divide5/1 -> Add1/2
  Add1/1 -> Add4/2, Memory3/1
  Memory3/1 -> Add1/1
  Memory4/1 -> Add2/1
  Add2/1 -> Add5/1, Memory4/1
  Divide6/1 -> Add2/2
  Memory5/1 -> Add3/1
  Add3/1 -> Add5/2, Memory5/1
  Divide8/1 -> Add3/2
  Vabc/1 -> abc to Alpha-Beta-Zero/1
  abc to Alpha-Beta-Zero/1 -> Demux2/1
  Memory/1 -> Sum/2
  Sum/1 -> Gain3/1, Switch2/3, Sum2/2
  Sum2/1 -> Switch2/1
  Constant2/1 -> Sum2/1
  Gain3/1 -> Switch2/2
  Constant3/1 -> Gain2/1
  Sum3/1 -> Initial_filter/1(original)
  Demux/1 -> Sum3/1
  Sum4/1 -> Initial_filter1/1(original)
  Demux/2 -> Sum4/1
  Demux3/1 -> Sum3/2
  Demux3/2 -> Sum4/2
  PQ/1 -> Gain7/1
  Initial_filter/1(filtered) -> [P]
  Initial_filter1/1(filtered) -> [Q]
  Initial_filter2/1(filtered) -> [dV]
  Initial_filter3/1(filtered) -> [dTheta]
  Complex to Magnitude-Angle/2 -> [Theta]
  Gain4/1 -> [Vmag]
  Complex to Magnitude-Angle/1 -> Gain4/1
  Real-Imag to Complex/1 -> Complex to Magnitude-Angle/1
  Demux2/1 -> Real-Imag to Complex/1
  Demux2/2 -> Real-Imag to Complex/2
  Gain2/1 -> Demux/1
  Gain7/1 -> Demux3/1
  Switch2/1 -> Sum5/1  "dTheta"
  Sum5/1 -> Initial_filter3/1(original)
  Constant/1 -> Sum5/2
  Add5/1 -> DEF/1
  Add4/1 -> Terminator/1

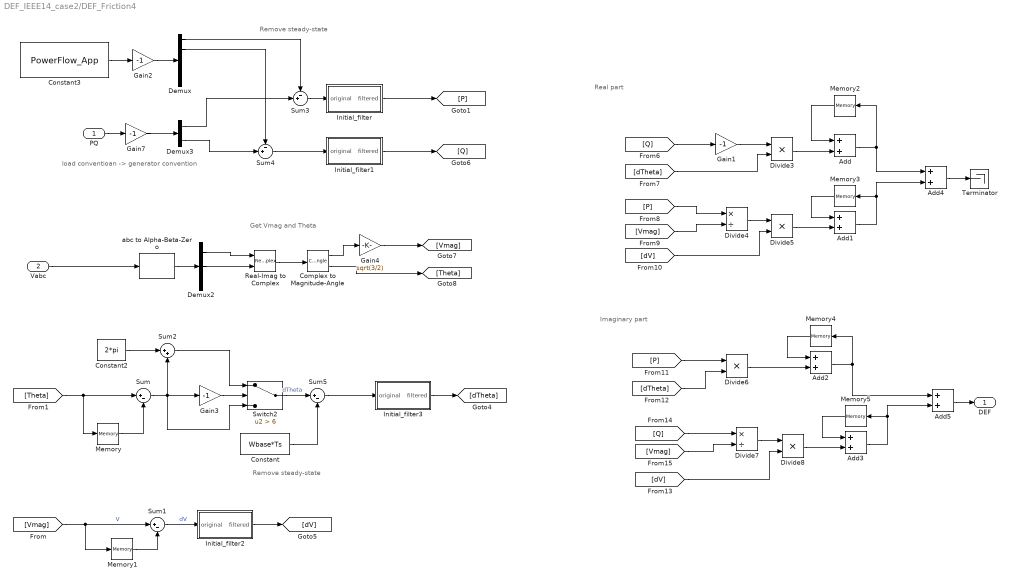
== system DEF_IEEE14_case2/DEF_Friction4 ==
  note: Real part
  note: Imaginary part
  note: load conventioan -> generator convention
  note: Remove steady-state
  note: Remove steady-state
  note: Get Vmag and Theta
  PQ : Inport
  Vabc : Inport  Port=2
  Add{,1..5} (6 alike) : Sum
  Complex to Magnitude-Angle : ComplexToMagnitudeAngle
  Constant : Constant  Value=Wbase*Ts
  Constant2 : Constant  Value=2*pi
  Constant3 : Constant  Value=PowerFlow_App
  Demux : Demux  Outputs=5
  Demux2 : Demux  Outputs=3
  Demux3 : Demux  Outputs=2
  Divide{3,5..6,8} (4 alike) : Product  Inputs=**
  Divide4 : Product  Inputs=*/
  Divide7 : Product  Inputs=*/
  Gain{1..3,7} (4 alike) : Gain  Gain=-1
  Gain4 : Gain  Gain=sqrt(3/2)
  Initial_filter : Subsystem
  Initial_filter1 : Subsystem
  Initial_filter2 : Subsystem
  Initial_filter3 : Subsystem
  Memory{,1..5} (6 alike) : Memory
  Real-Imag to Complex : RealImagToComplex
  Sum : Sum  Inputs=|+-
  Sum1 : Sum  Inputs=|+-
  Sum2 : Sum  Inputs=|++
  Sum3 : Sum  Inputs=-+|
  Sum4 : Sum  Inputs=-+|
  Sum5 : Sum  Inputs=|+-
  Switch2 : Switch  Criteria=u2 > Threshold  Threshold=6  SaturateOnIntegerOverflow=off  InputSameDT=off
  Terminator : Terminator
  abc to Alpha-Beta-Zero : spsabctoAlphaBetaZeroLib/abc to Alpha-Beta-Zero
  DEF : Outport
  wires:
  [Q] -> Divide7/1
  [Vmag] -> Divide4/2
  Divide3/1 -> Add/2
  [P] -> Divide4/1
  [Q] -> Gain1/1
  Gain1/1 -> Divide3/1
  [dTheta] -> Divide3/2
  [dV] -> Divide5/2
  [P] -> Divide6/1
  Divide4/1 -> Divide5/1
  [dTheta] -> Divide6/2
  [dV] -> Divide8/2
  Divide7/1 -> Divide8/1
  [Vmag] -> Divide7/2
  Memory1/1 -> Sum1/2
  [Vmag] -> Memory1/1, Sum1/1  "V"
  Sum1/1 -> Initial_filter2/1(original)  "dV"
  [Theta] -> Sum/1, Memory/1
  Add/1 -> Memory2/1, Add4/1
  Memory2/1 -> Add/1
  Divide5/1 -> Add1/2
  Add1/1 -> Add4/2, Memory3/1
  Memory3/1 -> Add1/1
  Memory4/1 -> Add2/1
  Add2/1 -> Add5/1, Memory4/1
  Divide6/1 -> Add2/2
  Memory5/1 -> Add3/1
  Add3/1 -> Add5/2, Memory5/1
  Divide8/1 -> Add3/2
  Vabc/1 -> abc to Alpha-Beta-Zero/1
  abc to Alpha-Beta-Zero/1 -> Demux2/1
  Memory/1 -> Sum/2
  Sum/1 -> Gain3/1, Switch2/3, Sum2/2
  Sum2/1 -> Switch2/1
  Constant2/1 -> Sum2/1
  Gain3/1 -> Switch2/2
  Constant3/1 -> Gain2/1
  Sum3/1 -> Initial_filter/1(original)
  Demux/1 -> Sum3/1
  Sum4/1 -> Initial_filter1/1(original)
  Demux/2 -> Sum4/1
  Demux3/1 -> Sum3/2
  Demux3/2 -> Sum4/2
  PQ/1 -> Gain7/1
  Initial_filter/1(filtered) -> [P]
  Initial_filter1/1(filtered) -> [Q]
  Initial_filter2/1(filtered) -> [dV]
  Initial_filter3/1(filtered) -> [dTheta]
  Complex to Magnitude-Angle/2 -> [Theta]
  Gain4/1 -> [Vmag]
  Complex to Magnitude-Angle/1 -> Gain4/1
  Real-Imag to Complex/1 -> Complex to Magnitude-Angle/1
  Demux2/1 -> Real-Imag to Complex/1
  Demux2/2 -> Real-Imag to Complex/2
  Gain2/1 -> Demux/1
  Gain7/1 -> Demux3/1
  Switch2/1 -> Sum5/1  "dTheta"
  Sum5/1 -> Initial_filter3/1(original)
  Constant/1 -> Sum5/2
  Add5/1 -> DEF/1
  Add4/1 -> Terminator/1

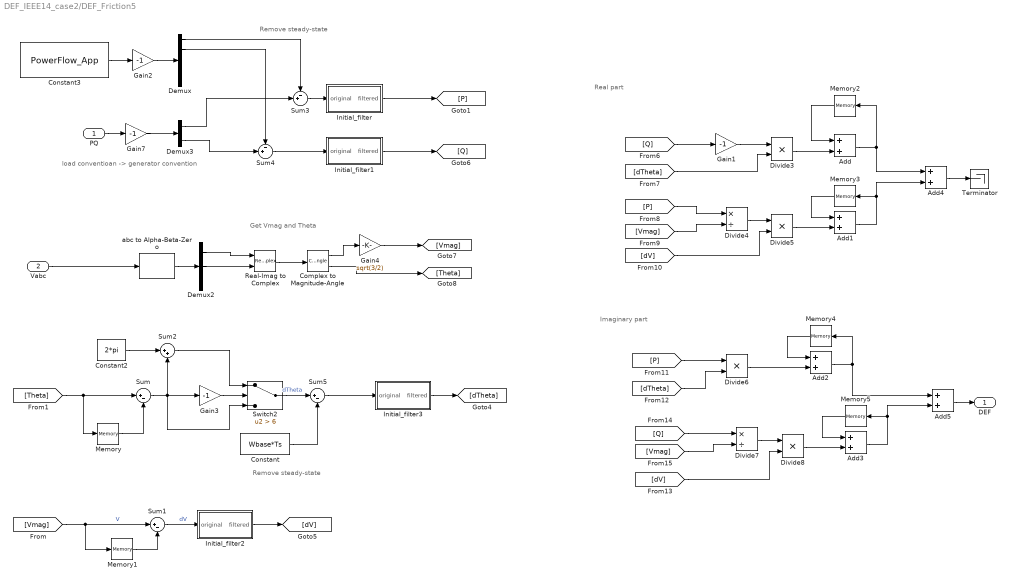
== system DEF_IEEE14_case2/DEF_Friction5 ==
  note: Real part
  note: Imaginary part
  note: load conventioan -> generator convention
  note: Remove steady-state
  note: Remove steady-state
  note: Get Vmag and Theta
  PQ : Inport
  Vabc : Inport  Port=2
  Add{,1..5} (6 alike) : Sum
  Complex to Magnitude-Angle : ComplexToMagnitudeAngle
  Constant : Constant  Value=Wbase*Ts
  Constant2 : Constant  Value=2*pi
  Constant3 : Constant  Value=PowerFlow_App
  Demux : Demux  Outputs=5
  Demux2 : Demux  Outputs=3
  Demux3 : Demux  Outputs=2
  Divide{3,5..6,8} (4 alike) : Product  Inputs=**
  Divide4 : Product  Inputs=*/
  Divide7 : Product  Inputs=*/
  Gain{1..3,7} (4 alike) : Gain  Gain=-1
  Gain4 : Gain  Gain=sqrt(3/2)
  Initial_filter : Subsystem
  Initial_filter1 : Subsystem
  Initial_filter2 : Subsystem
  Initial_filter3 : Subsystem
  Memory{,1..5} (6 alike) : Memory
  Real-Imag to Complex : RealImagToComplex
  Sum : Sum  Inputs=|+-
  Sum1 : Sum  Inputs=|+-
  Sum2 : Sum  Inputs=|++
  Sum3 : Sum  Inputs=-+|
  Sum4 : Sum  Inputs=-+|
  Sum5 : Sum  Inputs=|+-
  Switch2 : Switch  Criteria=u2 > Threshold  Threshold=6  SaturateOnIntegerOverflow=off  InputSameDT=off
  Terminator : Terminator
  abc to Alpha-Beta-Zero : spsabctoAlphaBetaZeroLib/abc to Alpha-Beta-Zero
  DEF : Outport
  wires:
  [Q] -> Divide7/1
  [Vmag] -> Divide4/2
  Divide3/1 -> Add/2
  [P] -> Divide4/1
  [Q] -> Gain1/1
  Gain1/1 -> Divide3/1
  [dTheta] -> Divide3/2
  [dV] -> Divide5/2
  [P] -> Divide6/1
  Divide4/1 -> Divide5/1
  [dTheta] -> Divide6/2
  [dV] -> Divide8/2
  Divide7/1 -> Divide8/1
  [Vmag] -> Divide7/2
  Memory1/1 -> Sum1/2
  [Vmag] -> Memory1/1, Sum1/1  "V"
  Sum1/1 -> Initial_filter2/1(original)  "dV"
  [Theta] -> Sum/1, Memory/1
  Add/1 -> Memory2/1, Add4/1
  Memory2/1 -> Add/1
  Divide5/1 -> Add1/2
  Add1/1 -> Add4/2, Memory3/1
  Memory3/1 -> Add1/1
  Memory4/1 -> Add2/1
  Add2/1 -> Add5/1, Memory4/1
  Divide6/1 -> Add2/2
  Memory5/1 -> Add3/1
  Add3/1 -> Add5/2, Memory5/1
  Divide8/1 -> Add3/2
  Vabc/1 -> abc to Alpha-Beta-Zero/1
  abc to Alpha-Beta-Zero/1 -> Demux2/1
  Memory/1 -> Sum/2
  Sum/1 -> Gain3/1, Switch2/3, Sum2/2
  Sum2/1 -> Switch2/1
  Constant2/1 -> Sum2/1
  Gain3/1 -> Switch2/2
  Constant3/1 -> Gain2/1
  Sum3/1 -> Initial_filter/1(original)
  Demux/1 -> Sum3/1
  Sum4/1 -> Initial_filter1/1(original)
  Demux/2 -> Sum4/1
  Demux3/1 -> Sum3/2
  Demux3/2 -> Sum4/2
  PQ/1 -> Gain7/1
  Initial_filter/1(filtered) -> [P]
  Initial_filter1/1(filtered) -> [Q]
  Initial_filter2/1(filtered) -> [dV]
  Initial_filter3/1(filtered) -> [dTheta]
  Complex to Magnitude-Angle/2 -> [Theta]
  Gain4/1 -> [Vmag]
  Complex to Magnitude-Angle/1 -> Gain4/1
  Real-Imag to Complex/1 -> Complex to Magnitude-Angle/1
  Demux2/1 -> Real-Imag to Complex/1
  Demux2/2 -> Real-Imag to Complex/2
  Gain2/1 -> Demux/1
  Gain7/1 -> Demux3/1
  Switch2/1 -> Sum5/1  "dTheta"
  Sum5/1 -> Initial_filter3/1(original)
  Constant/1 -> Sum5/2
  Add5/1 -> DEF/1
  Add4/1 -> Terminator/1

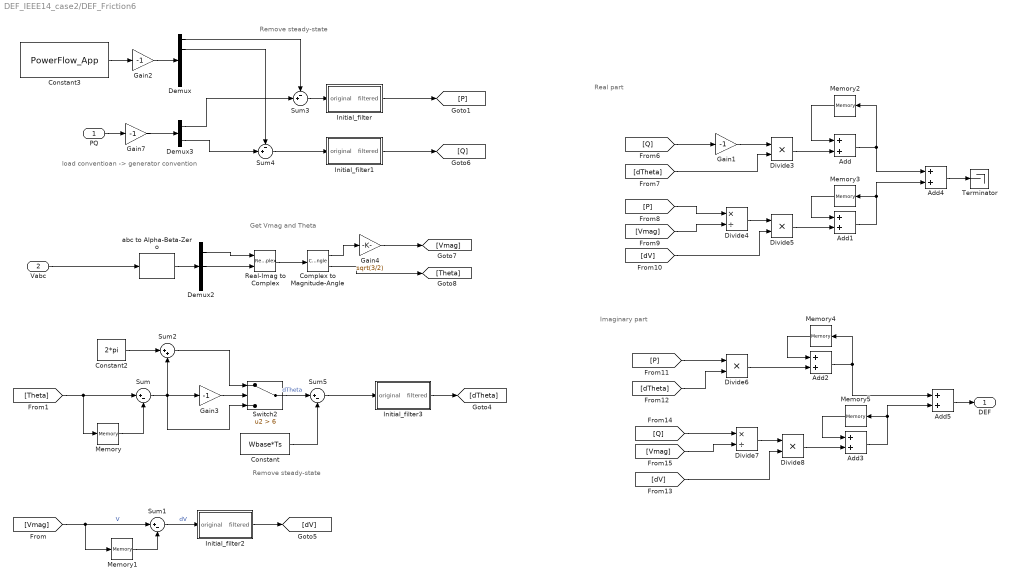
== system DEF_IEEE14_case2/DEF_Friction6 ==
  note: Real part
  note: Imaginary part
  note: load conventioan -> generator convention
  note: Remove steady-state
  note: Remove steady-state
  note: Get Vmag and Theta
  PQ : Inport
  Vabc : Inport  Port=2
  Add{,1..5} (6 alike) : Sum
  Complex to Magnitude-Angle : ComplexToMagnitudeAngle
  Constant : Constant  Value=Wbase*Ts
  Constant2 : Constant  Value=2*pi
  Constant3 : Constant  Value=PowerFlow_App
  Demux : Demux  Outputs=5
  Demux2 : Demux  Outputs=3
  Demux3 : Demux  Outputs=2
  Divide{3,5..6,8} (4 alike) : Product  Inputs=**
  Divide4 : Product  Inputs=*/
  Divide7 : Product  Inputs=*/
  Gain{1..3,7} (4 alike) : Gain  Gain=-1
  Gain4 : Gain  Gain=sqrt(3/2)
  Initial_filter : Subsystem
  Initial_filter1 : Subsystem
  Initial_filter2 : Subsystem
  Initial_filter3 : Subsystem
  Memory{,1..5} (6 alike) : Memory
  Real-Imag to Complex : RealImagToComplex
  Sum : Sum  Inputs=|+-
  Sum1 : Sum  Inputs=|+-
  Sum2 : Sum  Inputs=|++
  Sum3 : Sum  Inputs=-+|
  Sum4 : Sum  Inputs=-+|
  Sum5 : Sum  Inputs=|+-
  Switch2 : Switch  Criteria=u2 > Threshold  Threshold=6  SaturateOnIntegerOverflow=off  InputSameDT=off
  Terminator : Terminator
  abc to Alpha-Beta-Zero : spsabctoAlphaBetaZeroLib/abc to Alpha-Beta-Zero
  DEF : Outport
  wires:
  [Q] -> Divide7/1
  [Vmag] -> Divide4/2
  Divide3/1 -> Add/2
  [P] -> Divide4/1
  [Q] -> Gain1/1
  Gain1/1 -> Divide3/1
  [dTheta] -> Divide3/2
  [dV] -> Divide5/2
  [P] -> Divide6/1
  Divide4/1 -> Divide5/1
  [dTheta] -> Divide6/2
  [dV] -> Divide8/2
  Divide7/1 -> Divide8/1
  [Vmag] -> Divide7/2
  Memory1/1 -> Sum1/2
  [Vmag] -> Memory1/1, Sum1/1  "V"
  Sum1/1 -> Initial_filter2/1(original)  "dV"
  [Theta] -> Sum/1, Memory/1
  Add/1 -> Memory2/1, Add4/1
  Memory2/1 -> Add/1
  Divide5/1 -> Add1/2
  Add1/1 -> Add4/2, Memory3/1
  Memory3/1 -> Add1/1
  Memory4/1 -> Add2/1
  Add2/1 -> Add5/1, Memory4/1
  Divide6/1 -> Add2/2
  Memory5/1 -> Add3/1
  Add3/1 -> Add5/2, Memory5/1
  Divide8/1 -> Add3/2
  Vabc/1 -> abc to Alpha-Beta-Zero/1
  abc to Alpha-Beta-Zero/1 -> Demux2/1
  Memory/1 -> Sum/2
  Sum/1 -> Gain3/1, Switch2/3, Sum2/2
  Sum2/1 -> Switch2/1
  Constant2/1 -> Sum2/1
  Gain3/1 -> Switch2/2
  Constant3/1 -> Gain2/1
  Sum3/1 -> Initial_filter/1(original)
  Demux/1 -> Sum3/1
  Sum4/1 -> Initial_filter1/1(original)
  Demux/2 -> Sum4/1
  Demux3/1 -> Sum3/2
  Demux3/2 -> Sum4/2
  PQ/1 -> Gain7/1
  Initial_filter/1(filtered) -> [P]
  Initial_filter1/1(filtered) -> [Q]
  Initial_filter2/1(filtered) -> [dV]
  Initial_filter3/1(filtered) -> [dTheta]
  Complex to Magnitude-Angle/2 -> [Theta]
  Gain4/1 -> [Vmag]
  Complex to Magnitude-Angle/1 -> Gain4/1
  Real-Imag to Complex/1 -> Complex to Magnitude-Angle/1
  Demux2/1 -> Real-Imag to Complex/1
  Demux2/2 -> Real-Imag to Complex/2
  Gain2/1 -> Demux/1
  Gain7/1 -> Demux3/1
  Switch2/1 -> Sum5/1  "dTheta"
  Sum5/1 -> Initial_filter3/1(original)
  Constant/1 -> Sum5/2
  Add5/1 -> DEF/1
  Add4/1 -> Terminator/1

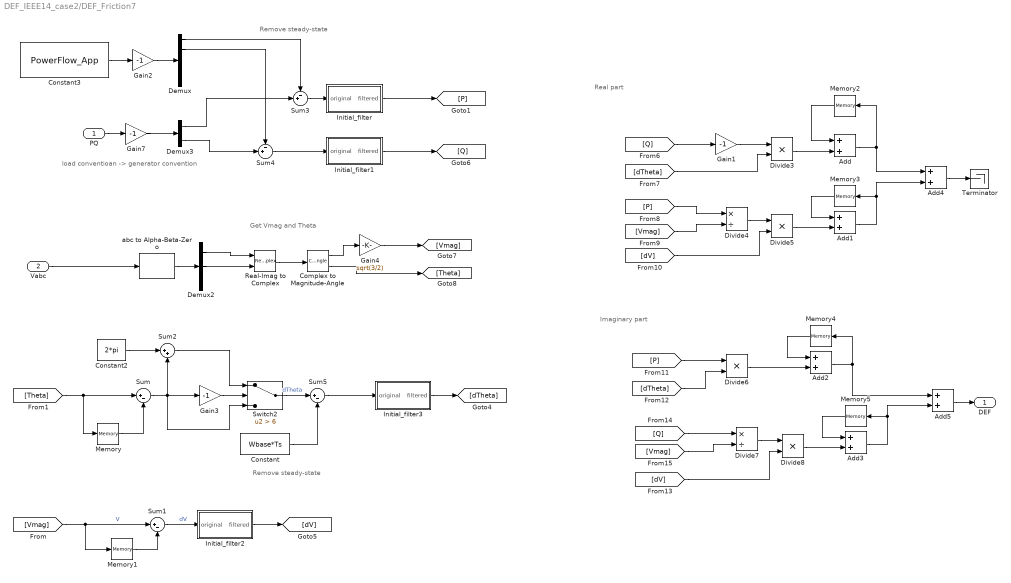
== system DEF_IEEE14_case2/DEF_Friction7 ==
  note: Real part
  note: Imaginary part
  note: load conventioan -> generator convention
  note: Remove steady-state
  note: Remove steady-state
  note: Get Vmag and Theta
  PQ : Inport
  Vabc : Inport  Port=2
  Add{,1..5} (6 alike) : Sum
  Complex to Magnitude-Angle : ComplexToMagnitudeAngle
  Constant : Constant  Value=Wbase*Ts
  Constant2 : Constant  Value=2*pi
  Constant3 : Constant  Value=PowerFlow_App
  Demux : Demux  Outputs=5
  Demux2 : Demux  Outputs=3
  Demux3 : Demux  Outputs=2
  Divide{3,5..6,8} (4 alike) : Product  Inputs=**
  Divide4 : Product  Inputs=*/
  Divide7 : Product  Inputs=*/
  Gain{1..3,7} (4 alike) : Gain  Gain=-1
  Gain4 : Gain  Gain=sqrt(3/2)
  Initial_filter : Subsystem
  Initial_filter1 : Subsystem
  Initial_filter2 : Subsystem
  Initial_filter3 : Subsystem
  Memory{,1..5} (6 alike) : Memory
  Real-Imag to Complex : RealImagToComplex
  Sum : Sum  Inputs=|+-
  Sum1 : Sum  Inputs=|+-
  Sum2 : Sum  Inputs=|++
  Sum3 : Sum  Inputs=-+|
  Sum4 : Sum  Inputs=-+|
  Sum5 : Sum  Inputs=|+-
  Switch2 : Switch  Criteria=u2 > Threshold  Threshold=6  SaturateOnIntegerOverflow=off  InputSameDT=off
  Terminator : Terminator
  abc to Alpha-Beta-Zero : spsabctoAlphaBetaZeroLib/abc to Alpha-Beta-Zero
  DEF : Outport
  wires:
  [Q] -> Divide7/1
  [Vmag] -> Divide4/2
  Divide3/1 -> Add/2
  [P] -> Divide4/1
  [Q] -> Gain1/1
  Gain1/1 -> Divide3/1
  [dTheta] -> Divide3/2
  [dV] -> Divide5/2
  [P] -> Divide6/1
  Divide4/1 -> Divide5/1
  [dTheta] -> Divide6/2
  [dV] -> Divide8/2
  Divide7/1 -> Divide8/1
  [Vmag] -> Divide7/2
  Memory1/1 -> Sum1/2
  [Vmag] -> Memory1/1, Sum1/1  "V"
  Sum1/1 -> Initial_filter2/1(original)  "dV"
  [Theta] -> Sum/1, Memory/1
  Add/1 -> Memory2/1, Add4/1
  Memory2/1 -> Add/1
  Divide5/1 -> Add1/2
  Add1/1 -> Add4/2, Memory3/1
  Memory3/1 -> Add1/1
  Memory4/1 -> Add2/1
  Add2/1 -> Add5/1, Memory4/1
  Divide6/1 -> Add2/2
  Memory5/1 -> Add3/1
  Add3/1 -> Add5/2, Memory5/1
  Divide8/1 -> Add3/2
  Vabc/1 -> abc to Alpha-Beta-Zero/1
  abc to Alpha-Beta-Zero/1 -> Demux2/1
  Memory/1 -> Sum/2
  Sum/1 -> Gain3/1, Switch2/3, Sum2/2
  Sum2/1 -> Switch2/1
  Constant2/1 -> Sum2/1
  Gain3/1 -> Switch2/2
  Constant3/1 -> Gain2/1
  Sum3/1 -> Initial_filter/1(original)
  Demux/1 -> Sum3/1
  Sum4/1 -> Initial_filter1/1(original)
  Demux/2 -> Sum4/1
  Demux3/1 -> Sum3/2
  Demux3/2 -> Sum4/2
  PQ/1 -> Gain7/1
  Initial_filter/1(filtered) -> [P]
  Initial_filter1/1(filtered) -> [Q]
  Initial_filter2/1(filtered) -> [dV]
  Initial_filter3/1(filtered) -> [dTheta]
  Complex to Magnitude-Angle/2 -> [Theta]
  Gain4/1 -> [Vmag]
  Complex to Magnitude-Angle/1 -> Gain4/1
  Real-Imag to Complex/1 -> Complex to Magnitude-Angle/1
  Demux2/1 -> Real-Imag to Complex/1
  Demux2/2 -> Real-Imag to Complex/2
  Gain2/1 -> Demux/1
  Gain7/1 -> Demux3/1
  Switch2/1 -> Sum5/1  "dTheta"
  Sum5/1 -> Initial_filter3/1(original)
  Constant/1 -> Sum5/2
  Add5/1 -> DEF/1
  Add4/1 -> Terminator/1
